simulink model "simu1"  (Simulink 7.1)
settings: Solver=ode45  StartTime=0.0  StopTime=10.0  RelTol=1e-3
undefined symbols (not defined in the file or in its folder): alpha1G, alpha2g, alpha3G, Ap, ap, Bp, bp, cp, K1G, K2G, Rn0, T1, Vc0
settings Model: Creator=knightofaccess  LastModifiedBy=ranjan

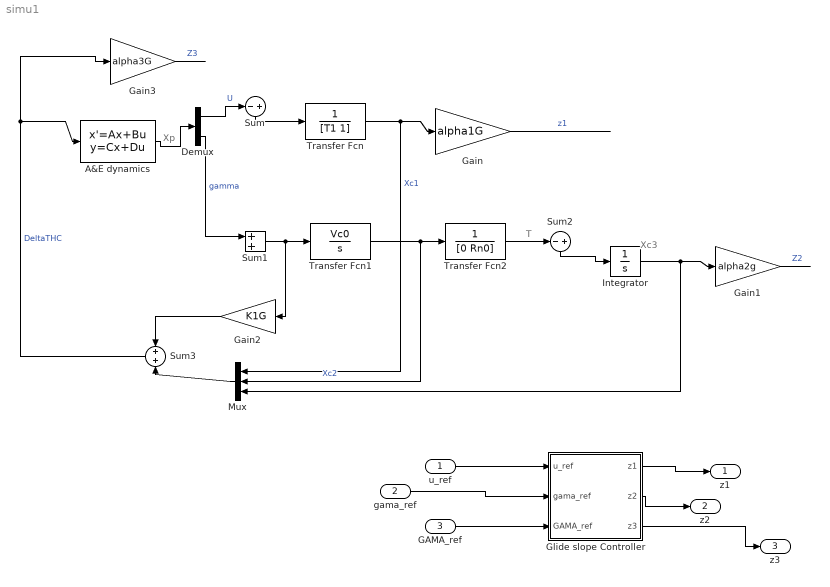
== system simu1 ==
  note: T
  note: Xc3
  note: Xp
  u_ref : Inport  OutDataType=sfix(16)  OutScaling=2^0
  gama_ref : Inport  Port=2  OutDataType=sfix(16)  OutScaling=2^0
  GAMA_ref : Inport  Port=3  OutDataType=sfix(16)  OutScaling=2^0
  A&E dynamics : StateSpace  A=Ap  B=Bp
  Demux : Demux  Outputs=2
  Gain : Gain  Gain=alpha1G  ParameterDataType=sfix(16)  ParameterScaling=2^0  OutDataType=sfix(16)  OutScaling=2^0
  Gain1 : Gain  Gain=alpha2g  ParameterDataType=sfix(16)  ParameterScaling=2^0  OutDataType=sfix(16)  OutScaling=2^0
  Gain2 : Gain  Orientation=left  Gain=K1G  ParameterDataType=sfix(16)  ParameterScaling=2^0  OutDataType=sfix(16)  OutScaling=2^0
  Gain3 : Gain  Gain=alpha3G  ParameterDataType=sfix(16)  ParameterScaling=2^0  OutDataType=sfix(16)  OutScaling=2^0
  Glide slope Controller : Subsystem
  Integrator : Integrator
  Mux : Mux  Orientation=left  Inputs=3
  Sum : Sum  Orientation=down  Inputs=-+  OutDataType=sfix(16)  OutScaling=2^0
  Sum1 : Sum  OutDataType=sfix(16)  OutScaling=2^0
  Sum2 : Sum  Orientation=down  Inputs=-+  OutDataType=sfix(16)  OutScaling=2^0
  Sum3 : Sum  Orientation=left  OutDataType=sfix(16)  OutScaling=2^0
  Transfer Fcn : TransferFcn  Denominator=[T1 1]
  Transfer Fcn1 : TransferFcn  Numerator=Vc0  Denominator=[1 0]
  Transfer Fcn2 : TransferFcn  Denominator=[0 Rn0]
  z1 : Outport  OutDataType=sfix(16)  OutScaling=2^0
  z2 : Outport  Port=2  OutDataType=sfix(16)  OutScaling=2^0
  z3 : Outport  Port=3  OutDataType=sfix(16)  OutScaling=2^0
  wires:
  A&E dynamics/1 -> Demux/1
  Demux/1 -> Sum/1  "U"
  Sum/1 -> Transfer Fcn/1
  Transfer Fcn/1 -> Gain/1, Mux/1  "Xc1"
  Gain/1 -> ?  "z1"
  Demux/2 -> Sum1/1  "gamma"
  ? -> Sum1/2  "gammaref"
  Sum1/1 -> Transfer Fcn1/1, Gain2/1
  Transfer Fcn1/1 -> Transfer Fcn2/1, Mux/2  "Xc2"
  Transfer Fcn2/1 -> Sum2/1
  Sum2/1 -> Integrator/1
  Integrator/1 -> Gain1/1, Mux/3
  Gain1/1 -> ?  "Z2"
  ? -> Sum2/2  "Tref"
  ? -> Sum/2  "Uref"
  Gain2/1 -> Sum3/1
  Mux/1 -> Sum3/2
  Sum3/1 -> Gain3/1, A&E dynamics/1  "DeltaTHC"
  Gain3/1 -> ?  "Z3"
  Glide slope Controller/1(z1) -> z1/1
  Glide slope Controller/2(z2) -> z2/1
  Glide slope Controller/3(z3) -> z3/1
  u_ref/1 -> Glide slope Controller/1(u_ref)
  gama_ref/1 -> Glide slope Controller/2(gama_ref)
  GAMA_ref/1 -> Glide slope Controller/3(GAMA_ref)

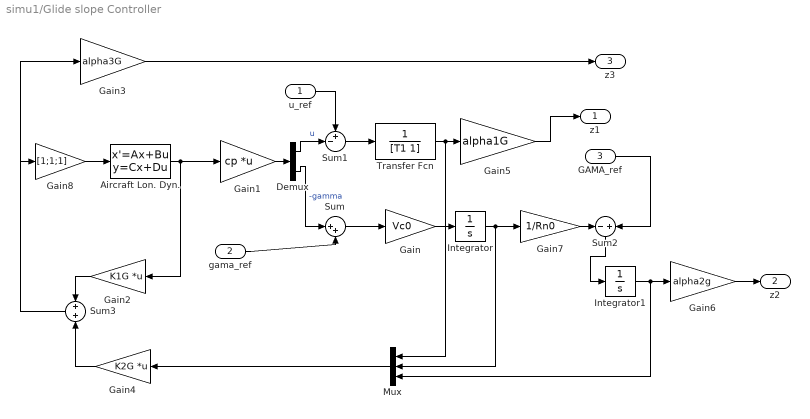
== system simu1/Glide slope Controller ==
  u_ref : Inport  OutDataType=sfix(16)  OutScaling=2^0
  gama_ref : Inport  Port=2  OutDataType=sfix(16)  OutScaling=2^0
  GAMA_ref : Inport  Port=3  OutDataType=sfix(16)  OutScaling=2^0
  Aircraft Lon. Dyn. : StateSpace  A=ap  B=bp  C=eye(4)  D=zeros(4,3)
  Demux : Demux  Outputs=2
  Gain : Gain  Gain=Vc0  ParameterDataType=sfix(16)  ParameterScaling=2^0  OutDataType=sfix(16)  OutScaling=2^0
  Gain1 : Gain  Gain=cp  Multiplication=Matrix(K*u)  ParameterDataType=sfix(16)  ParameterScaling=2^0  OutDataType=sfix(16)  OutScaling=2^0
  Gain2 : Gain  Orientation=left  Gain=K1G  Multiplication=Matrix(K*u)  ParameterDataType=sfix(16)  ParameterScaling=2^0  OutDataType=sfix(16)  OutScaling=2^0
  Gain3 : Gain  Gain=alpha3G  ParameterDataType=sfix(16)  ParameterScaling=2^0  OutDataType=sfix(16)  OutScaling=2^0
  Gain4 : Gain  Orientation=left  Gain=K2G  Multiplication=Matrix(K*u)  ParameterDataType=sfix(16)  ParameterScaling=2^0  OutDataType=sfix(16)  OutScaling=2^0
  Gain5 : Gain  Gain=alpha1G  ParameterDataType=sfix(16)  ParameterScaling=2^0  OutDataType=sfix(16)  OutScaling=2^0
  Gain6 : Gain  Gain=alpha2g  ParameterDataType=sfix(16)  ParameterScaling=2^0  OutDataType=sfix(16)  OutScaling=2^0
  Gain7 : Gain  Gain=1/Rn0  ParameterDataType=sfix(16)  ParameterScaling=2^0  OutDataType=sfix(16)  OutScaling=2^0
  Gain8 : Gain  Gain=[1;1;1]  ParameterDataType=sfix(16)  ParameterScaling=2^0  OutDataType=sfix(16)  OutScaling=2^0
  Integrator : Integrator
  Integrator1 : Integrator
  Mux : Mux  Orientation=left  Inputs=3
  Sum : Sum  Inputs=|++  OutDataType=sfix(16)  OutScaling=2^0
  Sum1 : Sum  Inputs=+-|  OutDataType=sfix(16)  OutScaling=2^0
  Sum2 : Sum  Orientation=down  Inputs=-+  OutDataType=sfix(16)  OutScaling=2^0
  Sum3 : Sum  Orientation=left  OutDataType=sfix(16)  OutScaling=2^0
  Transfer Fcn : TransferFcn  Denominator=[T1 1]
  z1 : Outport  OutDataType=sfix(16)  OutScaling=2^0
  z2 : Outport  Port=2  OutDataType=sfix(16)  OutScaling=2^0
  z3 : Outport  Port=3  OutDataType=sfix(16)  OutScaling=2^0
  wires:
  Gain/1 -> Integrator/1
  Sum/1 -> Gain/1
  Sum1/1 -> Transfer Fcn/1
  Aircraft Lon. Dyn./1 -> Gain1/1, Gain2/1
  Gain1/1 -> Demux/1
  Demux/1 -> Sum1/2  "u"
  Demux/2 -> Sum/1  "-gamma"
  Gain2/1 -> Sum3/1
  Sum3/1 -> Gain3/1, Gain8/1
  Mux/1 -> Gain4/1
  Gain4/1 -> Sum3/2
  Integrator/1 -> Mux/2, Gain7/1
  Transfer Fcn/1 -> Mux/1, Gain5/1
  Gain7/1 -> Sum2/1
  Sum2/1 -> Integrator1/1
  Integrator1/1 -> Gain6/1, Mux/3
  u_ref/1 -> Sum1/1
  gama_ref/1 -> Sum/2
  GAMA_ref/1 -> Sum2/2
  Gain5/1 -> z1/1
  Gain6/1 -> z2/1
  Gain3/1 -> z3/1
  Gain8/1 -> Aircraft Lon. Dyn./1
